simulink model "deTremblay1992Model"  (R2022a)
settings: Solver=VariableStepAuto  StartTime=0.0  StopTime=240  RelTol=1e-3
model workspace (MAT data in the model file):
  Q_in = [0.12271780758; 0.123470790595; 0.124228393831; 0.124990645638; 0.125757574538; 0.12652920923; 0.127305578587]
  Sig = Simulink.Signal
  Sig.DataType = 'auto'
  Sig.Dimensions = -1
  Sig.DimensionsMode = 'auto'
  Sig.Complexity = 'auto'
  Sig.SampleTime = -1
  Sig.SamplingMode = 'auto'
  x0 = [0.2; 200000000; 200000000; 25.1; 5.01; 0; 0; 100; 0; 0; 0; 0; 0; 0; 0; 0]
libraries: simulink x2
settings Model: Creator=tomok  LastModifiedBy=tomok
settings DataIOCC: ReturnWorkspaceOutputsName=SimLog

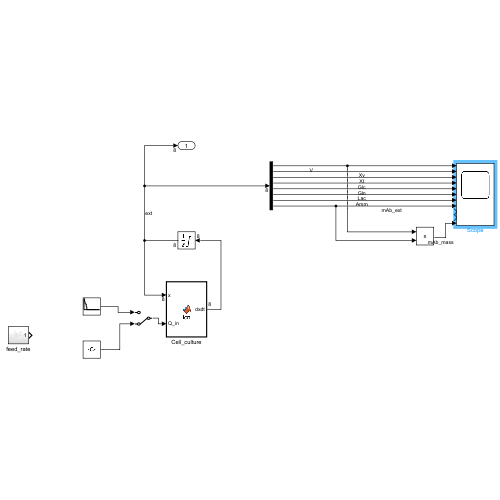
[thumbnail: Simulink's stored preview of the top-level diagram]
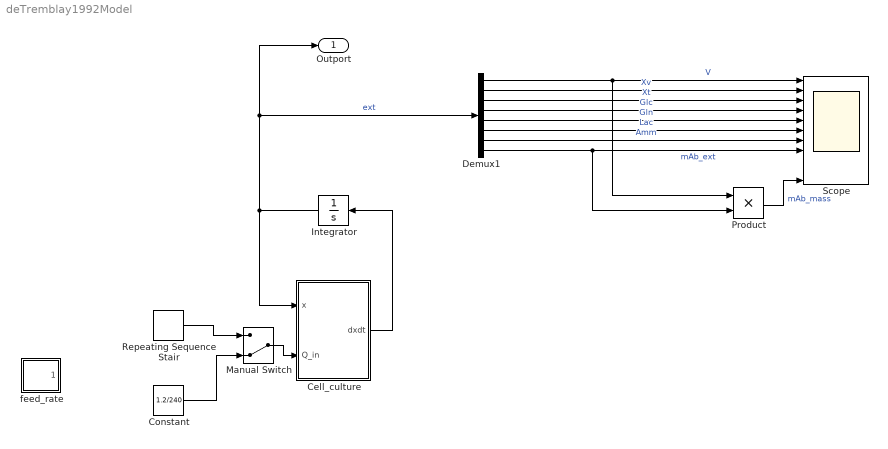
== system deTremblay1992Model ==
  Cell_culture : MATLAB Function  TreatAsAtomicUnit=on
  Constant : Constant  Value=1.2/240
  Demux1 : Demux  Outputs=8
  Integrator : Integrator  InitialCondition=[0.8;2E+8;2E+8;25;4;0;0;0]  LimitOutput=on  LowerSaturationLimit=0
  Manual Switch : ManualSwitch  CurrentSetting=0
  Product : Product
  Repeating Sequence Stair : simulink/Sources/Repeating Sequence Stair  OutValues=Info_true.MVopt  tsamp=12  OutMin=[]  OutMax=[]  OutDataTypeStr=double  OutputDataTypeScalingMode=double  OutDataType=fixdt(0,8)  ConRadixGroup=Best Precision: Vector-wise  OutScaling=2^-12
  Scope : Scope  NumInputPorts=11
  feed_rate : Subsystem
  Outport : Outport  SampleTime=12
  wires:
  Cell_culture/1(dxdt) -> Integrator/1
  Integrator/1 -> Outport/1, Demux1/1, Cell_culture/1(x)  "ext"
  Demux1/1 -> Product/1, Scope/1  "V"
  Demux1/2 -> Scope/2  "Xv"
  Demux1/3 -> Scope/3  "Xt"
  Demux1/4 -> Scope/4  "Glc"
  Demux1/5 -> Scope/5  "Gln"
  Demux1/6 -> Scope/6  "Lac"
  Demux1/7 -> Scope/7  "Amm"
  Demux1/8 -> Product/2, Scope/8  "mAb_ext"
  Manual Switch/1 -> Cell_culture/2(Q_in)
  Constant/1 -> Manual Switch/2
  Product/1 -> Scope/11  "mAb_mass"
  Repeating Sequence Stair/1 -> Manual Switch/1

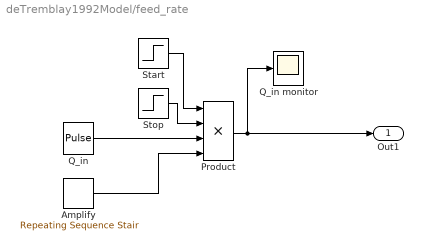
== system deTremblay1992Model/feed_rate ==
  Amplify : simulink/Sources/Repeating Sequence Stair  OutValues=Q_in  tsamp=24  OutMin=[]  OutMax=[]  OutDataTypeStr=double  OutputDataTypeScalingMode=double  OutDataType=fixdt(0,8)  ConRadixGroup=Best Precision: Vector-wise  OutScaling=2^-12
  Product : Product  Inputs=4
  Q_in : DiscretePulseGenerator  PulseType=Time based  Period=24  PulseWidth=1/24  PhaseDelay=12
  Q_in monitor : Scope
  Start : Step  SampleTime=0
  Stop : Step  Time=169  Before=1  After=0  SampleTime=0
  Out1 : Outport
  wires:
  Stop/1 -> Product/2
  Start/1 -> Product/1
  Product/1 -> Q_in monitor/1, Out1/1
  Q_in/1 -> Product/3
  Amplify/1 -> Product/4

== matlab function deTremblay1992Model/Cell_culture ==
  data: dxdt output; x input; Q_in input
function dxdt = fcn(x,Q_in)
dxdt = deTremblay1992StateFcn(x,Q_in);
end
